simulink model "kabdalproject6"  (Simulink 7.7)
settings: Solver=ode23tb  StartTime=0.0  StopTime=1.0  RelTol=1e-3
libraries: powerlib x4
settings Model: Creator=Shailesh  LastModifiedBy=Shailesh
settings OptimizationCC: InlineInvariantSignals=on  InitFltsAndDblsToZero=on
settings DebuggingCC: SaveWithParameterizedLinksMsg=none  SignalResolutionControl=TryResolveAllWithWarning  MultiTaskDSMMsg=warning  MultiTaskCondExecSysMsg=none  StrictBusMsg=None
settings RTWCC: IncludeERTFirstTime=on
settings GRTTargetCC: TargetFcnLib=ansi_tfl_tmw.mat

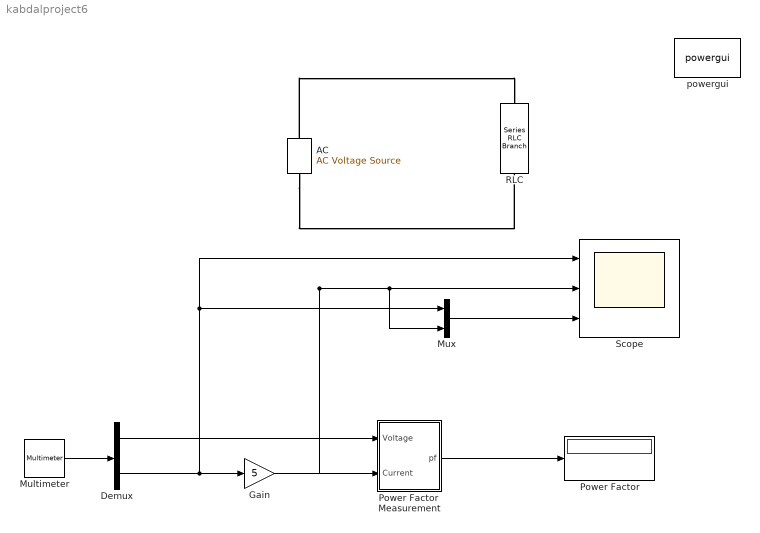
== system kabdalproject6 ==
  " RLC" : powerlib/Elements/Series RLC Branch  PhysicalDomain=powersysdomain  SubClassName=unknown  LeftPortType=p1  RightPortType=p1  LConnTagsString=__new0  RConnTagsString=__new0  BranchType=RLC  Resistance=3  Inductance=.3  SetiL0=off  InitialCurrent=0  Capacitance=inf  Setx0=off  InitialVoltage=0  Measurements=Branch current
  "AC " : powerlib/Electrical Sources/AC Voltage Source  SystemSampleTime=-1  Amplitude=5  Phase=0  Frequency=5  SampleTime=0  Measurements=Voltage
      link override Goto: GotoTag=tp223391
  Demux : Demux  Outputs=2
  Gain : Gain  Gain=5
  Multimeter : powerlib/Measurements/Multimeter  SystemSampleTime=-1  PhasorSimulation=off  OutputType=Complex  sel=[1 2]  L=2  Gain=[1 1]  yselected="{'Usrc: AC Voltage Source','Ib:  RLC'};"  PSBOutputType=1  PSBequivalent=0  AxesSetting=[0,0.1,-100,100]  Display=0  SavedBlockNames=-11
  Mux : Mux  Inputs=2
  Power Factor : Display
  Power Factor  Measurement : Subsystem
  Scope : Scope  NumInputPorts=3
      settings: TickLabels=on  TimeRange=1  YMin=-5~-0.1~-5  YMax=5~0.1~5
  powergui : powerlib/powergui  Priority=1  SystemSampleTime=-1  SimulationMode=Continuous  SampleTime=50e-6  frequency=60  SPID=off  DisableSnubberDevices=off  DisableRonSwitches=off  DisableVfSwitches=off  SwTol=0  Interpol=off  DisplayEquations=off  FunctionMessages=off  frequencyindice=5  Pbase=100e6  ErrMax=1e-4  Iterations=50  UnitsV=kV  UnitsW=MW  echomessages=off  HookPort=off  EnableUseOfTLC=off  x0status=blocks  RestoreLinks=warning  ResistiveCurrentMeasurement=off  Ylog=off  Xlog=on  ShowGrid=off  save=off  variable=ZData  ZoomFFT=off  StartTime=0.0  cycles=1  DisplayStyle=1  FreqAxis=off  MaxFrequency=1000  frequencyindicesteady=1  display=off  methode=off
  wires:
  Power Factor  Measurement/1(pf) -> Power Factor/1
  Mux/1 -> Scope/3
  Gain/1 -> Power Factor  Measurement/2(Current), Mux/2, Scope/2
  Multimeter/1 -> Demux/1
  Demux/1 -> Power Factor  Measurement/1(Voltage)
  Demux/2 -> Gain/1, Mux/1, Scope/1
  connections:
  "AC "/LConn1 -- " RLC"/RConn1
  "AC "/RConn1 -- " RLC"/LConn1

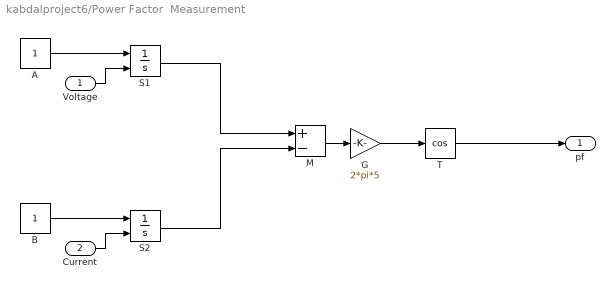
== system kabdalproject6/Power Factor  Measurement ==
  Voltage : Inport
  Current : Inport  Port=2
  A : Constant
  B : Constant
  G : Gain  Gain=2*pi*5
  M : Sum  Inputs=+-
  S1 : Integrator  ExternalReset=falling
  S2 : Integrator  ExternalReset=falling
  T : Trigonometry  Operator=cos
  pf : Outport
  wires:
  A/1 -> S1/1
  B/1 -> S2/1
  S1/1 -> M/1
  S2/1 -> M/2
  Voltage/1 -> S1/2
  Current/1 -> S2/2
  M/1 -> G/1
  G/1 -> T/1
  T/1 -> pf/1
